simulink model "SIL"  (R2025b)
settings: Solver=FixedStepDiscrete  StartTime=0.0  StopTime=inf  FixedStep=0.01  RelTol=1e-3
libraries: dspnetwork x1
settings Model: NumberOfSteps=10  Creator=Gabriel  LastModifiedBy=henri
settings SFSimCC: SimCustomInitializer=SS_App_Init();  SimUserIncludeDirs=..\..\include
settings SFSimCC: SimCustomHeaderCode=|
  | #include "ss_app.h"
  | 
  | #include "ss_input_proc.h"
  | 
  | #include "ss_operation.h"
  | 
  | #include "ss_types.h"
  | 
  | #include "ss_calib.h"
  | 
  | #include "ss_timer.h"
  | 
  | #include "ss_inhibit_safety_conditions.h"
  | 
  | #include "co2.h"
  | 
  | #include "ss_fuel.h"
  | 
  | #include "ss_control.h"
settings SFSimCC: SimUserSources=|
  | ..\..\src\ss_operation.c
  | 
  | ..\..\src\ss_input_proc.c
  | 
  | ..\..\src\ss_app.c
  | 
  | ..\..\src\timer.c
  | 
  | ..\..\src\ss_inhibit_safety_conditions.c
  | 
  | ..\..\src\co2.c
  | 
  | ..\..\src\ss_control.c
  | 
  | ..\..\src\ss_fuel.c

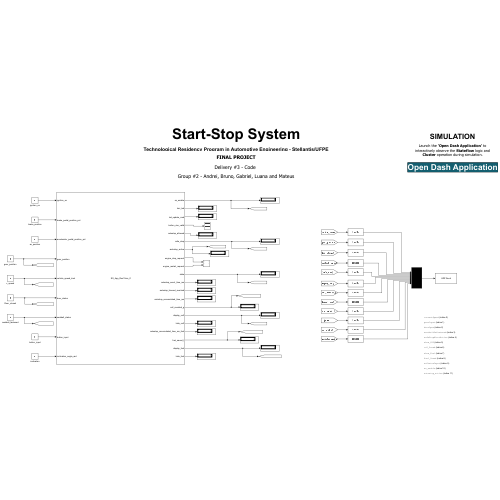
[thumbnail: Simulink's stored preview of the top-level diagram]
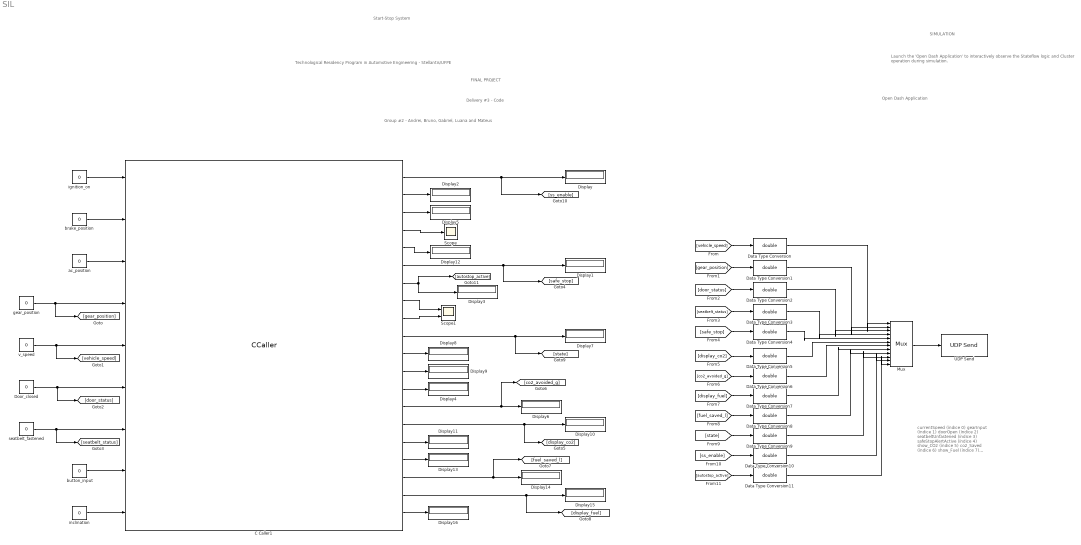
== system SIL ==
  note: currentSpeed (índice 0)
      | gearInput (índice 1)
      | doorOpen (índice 2)
      | seatbeltUnfastened (índice 3)
      | safeStopAlertActive (índice 4)
      | show_CO2 (índice 5)
      | co2_Saved (índice 6)
      | show_Fuel (índice 7)
      | fuel_Saved (índice 8)
      | ssStatusInput (índice 9)
      | ss_enable (índice 10)
      |
      | autostop_active (índice 11)
  note: Open Dash Application
  note: Technological Residency Program in Automotive Engineering - Stellantis/UFPE
  note: Start-Stop System
  note: FINAL PROJECT
  note: Group #2 - Andrei, Bruno, Gabriel, Luana and Mateus
  note: Delivery #3 - Code
  note: SIMULATION
  note: Launch the 'Open Dash Application' to interactively observe the Stateflow logic and Cluster operation during simulation.
  C Caller1 : CCaller  FunctionName=SS_App_Run10ms_If  PortSpecificationStruct="%)30     .    ^#,   8    (     @         %    \"    !T    !     0         %  0 \"0    $    _    07)G3F%M90  4&]R=$YA;64 4V-O<&4     26YD97@     5'EP90      4VEZ90      27-';&]B86P   X   !     !@    @    $          4    (     0    L    !         !     +    :6=N:71I;VY?;VX       X   !     !@    @    $          4    (     0    L    !         !     +    :6=N:71I;VY?;VX       X    X    !@    @    $     ...(+17556 chars)"  SampleTime=0.01
  Data Type Conversion{,1..11} (12 alike) : DataTypeConversion  OutDataTypeStr=double  SaturateOnIntegerOverflow=off  RndMeth=Floor
  Display{,1..16} (17 alike) : Display
  Door_closed : Constant  Value=0  OutDataTypeStr=boolean
  Mux : Mux  Inputs=12
  Scope : Scope
      settings: ActiveDisplayYMinimum=-1.3720535825056084  ActiveDisplayYMaximum=4.2527611164993893
  Scope1 : Scope  NumInputPorts=2
      settings: ActiveDisplayYMinimum=-1.3720535825056084  ActiveDisplayYMaximum=4.2527611164993893
  UDP Send : dspnetwork/UDP Send  remoteURL='127.0.0.1'  remotePort=55000  localURL='0.0.0.0'  localPortSource=Automatically determine  localPort=-1  sendBufferSize=8192  sampletime=-1  blockPlatform=[]  separateLengthPort=0
      settings: LibrarySourceBlock=dspsnks4/UDP Send
  ac_position : Constant  Value=0  OutDataTypeStr=single
  brake_position : Constant  Value=0  OutDataTypeStr=single
  button_input : Constant  Value=0  OutDataTypeStr=boolean
  gear_position : Constant  Value=0  OutDataTypeStr=int32
  ignition_on : Constant  Value=0  OutDataTypeStr=boolean
  inclination : Constant  Value=0  OutDataTypeStr=single
  seatbelt_fastened : Constant  Value=0  OutDataTypeStr=boolean
  v_speed : Constant  Value=0  OutDataTypeStr=single
  wires:
  ignition_on/1 -> C Caller1/1
  C Caller1/1 -> [ss_enable], Display/1
  C Caller1/2 -> Display2/1
  C Caller1/4 -> Scope/1
  C Caller1/6 -> [safe_stop], Display1/1
  C Caller1/3 -> Display5/1
  C Caller1/7 -> Display3/1, [autostop_active]
  C Caller1/8 -> Scope1/1
  C Caller1/9 -> Scope1/2
  C Caller1/10 -> [state], Display7/1
  C Caller1/11 -> Display8/1
  C Caller1/12 -> Display9/1
  brake_position/1 -> C Caller1/2
  ac_position/1 -> C Caller1/3
  gear_position/1 -> [gear_position], C Caller1/4
  v_speed/1 -> [vehicle_speed], C Caller1/5
  Door_closed/1 -> [door_status], C Caller1/6
  seatbelt_fastened/1 -> [seatbelt_status], C Caller1/7
  button_input/1 -> C Caller1/8
  inclination/1 -> C Caller1/9
  C Caller1/13 -> Display4/1
  C Caller1/14 -> [co2_avoided_g], Display6/1
  C Caller1/15 -> [display_co2], Display10/1
  C Caller1/16 -> Display11/1
  C Caller1/5 -> Display12/1
  C Caller1/17 -> Display13/1
  C Caller1/18 -> [fuel_saved_l], Display14/1
  C Caller1/19 -> [display_fuel], Display15/1
  C Caller1/20 -> Display16/1
  [vehicle_speed] -> Data Type Conversion/1
  [gear_position] -> Data Type Conversion1/1
  [door_status] -> Data Type Conversion2/1
  [seatbelt_status] -> Data Type Conversion3/1
  [safe_stop] -> Data Type Conversion4/1
  [display_co2] -> Data Type Conversion5/1
  [co2_avoided_g] -> Data Type Conversion6/1
  [display_fuel] -> Data Type Conversion7/1
  [fuel_saved_l] -> Data Type Conversion8/1
  [state] -> Data Type Conversion9/1
  Data Type Conversion/1 -> Mux/1
  Data Type Conversion1/1 -> Mux/2
  Data Type Conversion2/1 -> Mux/3
  Data Type Conversion3/1 -> Mux/4
  Data Type Conversion4/1 -> Mux/5
  Data Type Conversion5/1 -> Mux/6
  Data Type Conversion6/1 -> Mux/7
  Data Type Conversion7/1 -> Mux/8
  Data Type Conversion8/1 -> Mux/9
  Data Type Conversion9/1 -> Mux/10
  Mux/1 -> UDP Send/1
  Data Type Conversion10/1 -> Mux/11
  [ss_enable] -> Data Type Conversion10/1
  Data Type Conversion11/1 -> Mux/12
  [autostop_active] -> Data Type Conversion11/1
